simulink model "b6_formation"  (R2021b)
settings: Solver=FixedStepAuto  StartTime=0.0  StopTime=inf  FixedStep=sampleTime  RelTol=1e-3
PreLoadFcn:
  | % Simulation parameters
  | %load exampleMap
  | 
  | % Lidar parameters
  | sensorOffset = [0,0];
  | scanAngles = -pi/2:pi/6:pi/2;
  | maxRange = 0.3;
InitFcn:
  | sampleTime = 0.05;
  | nMedianSize=3;
  | % Robot parameters
  | wheelRadius = 0.0335;
  | robotRadius = 0.116/2;
  | 
  | %角速度坐标
  | ks=1;
  | 
  | % Lidar parameters
  | sensorOffset = [0,0];
  | scanAngles = -pi:pi/36:pi;
  | maxRange = 0.2;
  | 
  | %车初始位置
  | init_pose_1=[1  1.3  pi/2]';
  | init_pose_2=[0.85 1  pi/2]';
  | init_pose_3=[1.15 1  pi/2]';
  | init_pose_4=[0.7  0.7 pi/2]';
  | init_pose_5=[1  0.7 pi/2]';
  | init_pose_6=[1.3 0.7  pi/2]';
  | 
  | %pp算法性能参数
  | Vd_pp=0.2;
  | Wd_pp=pi;
  | dist_pp=0.2;
  | GoalRadius=0.1;
  | numSector=180;
  | rangeDis=[0.1,maxRange];
  | thresholds=[1/360 1/36];
  | safetyDis=0.2;
  | minimumTurningRadius=0.5*robotRadius;
  | recovery_w=0.05;
undefined symbols (not defined in the file): Angular, DiscIntNeverNeededParam, Linear, Pose, Twist
libraries: robotlib x42, dspstat3 x18, mobileRoboticsLib x7, robotmobilelib x6, robotalgslib x6
(part 1 of 5)
settings Model: Creator=FCS  LastModifiedBy=FCS

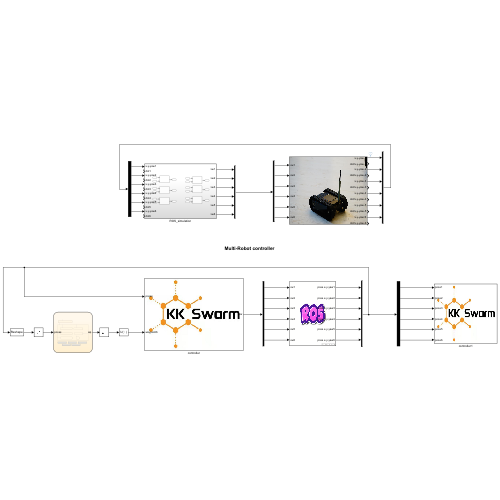
[thumbnail: Simulink's stored preview of the top-level diagram]
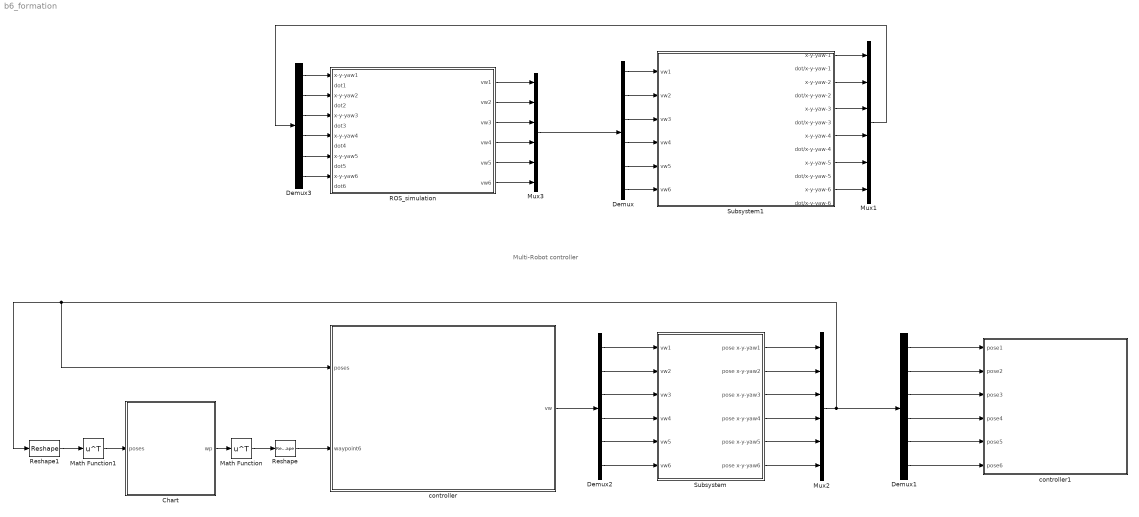
== system b6_formation ==
  note: Multi-Robot controller
  Chart : Stateflow chart  TreatAsAtomicUnit=on
  Demux{,1..3} (4 alike) : Demux  Outputs=6
  Math Function : Math  Operator=transpose  SaturateOnIntegerOverflow=on
  Math Function1 : Math  Operator=transpose  SaturateOnIntegerOverflow=on
  Mux1 : Mux  Inputs=6
  Mux2 : Mux  Inputs=6
  Mux3 : Mux  Inputs=6
  ROS_simulation : Subsystem
  Reshape : Reshape
  Reshape1 : Reshape  OutputDimensionality=Customize  OutputDimensions=[3,6]
  Subsystem : Subsystem
      mask Display: image('$imagefile'); % 使用工具条上的 "编辑图像" 进行更改。
  Subsystem1 : Subsystem
      mask Display: image('$imagefile'); % 使用工具条上的 "编辑图像" 进行更改。
  controller : Subsystem
      mask Display: image('$imagefile'); % 使用工具条上的 "编辑图像" 进行更改。
  controller1 : Subsystem
      mask Display: image('$imagefile'); % 使用工具条上的 "编辑图像" 进行更改。
  wires:
  Demux3/5 -> ROS_simulation/9(x-y-yaw5)
  Demux/3 -> Subsystem1/3(vw3)
  ROS_simulation/2(vw2) -> Mux3/2
  Demux3/1 -> ROS_simulation/1(x-y-yaw1)
  Subsystem1/9(x-y-yaw-5) -> Mux1/5
  Demux/2 -> Subsystem1/2(vw2)
  Demux/5 -> Subsystem1/5(vw5)
  Demux3/2 -> ROS_simulation/3(x-y-yaw2)
  Mux1/1 -> Demux3/1
  Subsystem1/1(x-y-yaw-1) -> Mux1/1
  ROS_simulation/5(vw5) -> Mux3/5
  Subsystem1/5(x-y-yaw-3) -> Mux1/3
  ROS_simulation/3(vw3) -> Mux3/3
  Subsystem1/7(x-y-yaw-4) -> Mux1/4
  Subsystem1/3(x-y-yaw-2) -> Mux1/2
  Demux3/4 -> ROS_simulation/7(x-y-yaw4)
  ROS_simulation/6(vw6) -> Mux3/6
  Demux/4 -> Subsystem1/4(vw4)
  ROS_simulation/4(vw4) -> Mux3/4
  Demux/1 -> Subsystem1/1(vw1)
  ROS_simulation/1(vw1) -> Mux3/1
  Subsystem1/11(x-y-yaw-6) -> Mux1/6
  Demux/6 -> Subsystem1/6(vw6)
  Mux3/1 -> Demux/1
  Demux3/3 -> ROS_simulation/5(x-y-yaw3)
  Demux3/6 -> ROS_simulation/11(x-y-yaw6)
  Subsystem/3(pose x-y-yaw3) -> Mux2/3
  Subsystem/6(pose x-y-yaw6) -> Mux2/6
  Subsystem/1(pose x-y-yaw1) -> Mux2/1
  Demux2/1 -> Subsystem/1(vw1)
  Demux2/2 -> Subsystem/2(vw2)
  Demux2/6 -> Subsystem/6(vw6)
  Demux2/4 -> Subsystem/4(vw4)
  Subsystem/4(pose x-y-yaw4) -> Mux2/4
  Demux2/3 -> Subsystem/3(vw3)
  Subsystem/2(pose x-y-yaw2) -> Mux2/2
  Subsystem/5(pose x-y-yaw5) -> Mux2/5
  Demux2/5 -> Subsystem/5(vw5)
  controller/1(vw) -> Demux2/1
  Chart/1(wp) -> Math Function/1
  Math Function/1 -> Reshape/1
  Reshape/1 -> controller/2(waypoint6)
  Reshape1/1 -> Math Function1/1
  Math Function1/1 -> Chart/1(poses)
  Mux2/1 -> Reshape1/1, controller/1(poses), Demux1/1
  Demux1/1 -> controller1/1(pose1)
  Demux1/2 -> controller1/2(pose2)
  Demux1/3 -> controller1/3(pose3)
  Demux1/4 -> controller1/4(pose4)
  Demux1/5 -> controller1/5(pose5)
  Demux1/6 -> controller1/6(pose6)

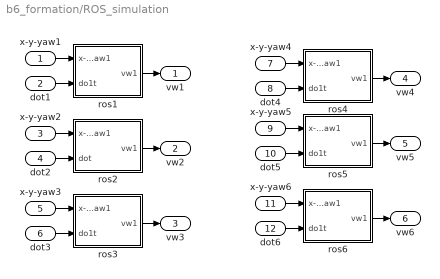
== system b6_formation/ROS_simulation ==
  x-y-yaw1 : Inport
  dot1 : Inport  Port=2
  x-y-yaw2 : Inport  Port=3
  dot2 : Inport  Port=4
  x-y-yaw3 : Inport  Port=5
  dot3 : Inport  Port=6
  x-y-yaw4 : Inport  Port=7
  dot4 : Inport  Port=8
  x-y-yaw5 : Inport  Port=9
  dot5 : Inport  Port=10
  x-y-yaw6 : Inport  Port=11
  dot6 : Inport  Port=12
  ros1 : Subsystem
  ros2 : Subsystem
  ros3 : Subsystem
  ros4 : Subsystem
  ros5 : Subsystem
  ros6 : Subsystem
  vw1 : Outport
  vw2 : Outport  Port=2
  vw3 : Outport  Port=3
  vw4 : Outport  Port=4
  vw5 : Outport  Port=5
  vw6 : Outport  Port=6
  wires:
  ros5/1(vw1) -> vw5/1
  ros2/1(vw1) -> vw2/1
  dot3/1 -> ros3/2(do1t)
  x-y-yaw5/1 -> ros5/1(x-y-yaw1)
  ros3/1(vw1) -> vw3/1
  dot2/1 -> ros2/2(dot)
  x-y-yaw2/1 -> ros2/1(x-y-yaw1)
  dot5/1 -> ros5/2(do1t)
  dot4/1 -> ros4/2(do1t)
  x-y-yaw4/1 -> ros4/1(x-y-yaw1)
  ros4/1(vw1) -> vw4/1
  x-y-yaw3/1 -> ros3/1(x-y-yaw1)
  dot6/1 -> ros6/2(do1t)
  x-y-yaw6/1 -> ros6/1(x-y-yaw1)
  dot1/1 -> ros1/2(do1t)
  ros6/1(vw1) -> vw6/1
  x-y-yaw1/1 -> ros1/1(x-y-yaw1)
  ros1/1(vw1) -> vw1/1

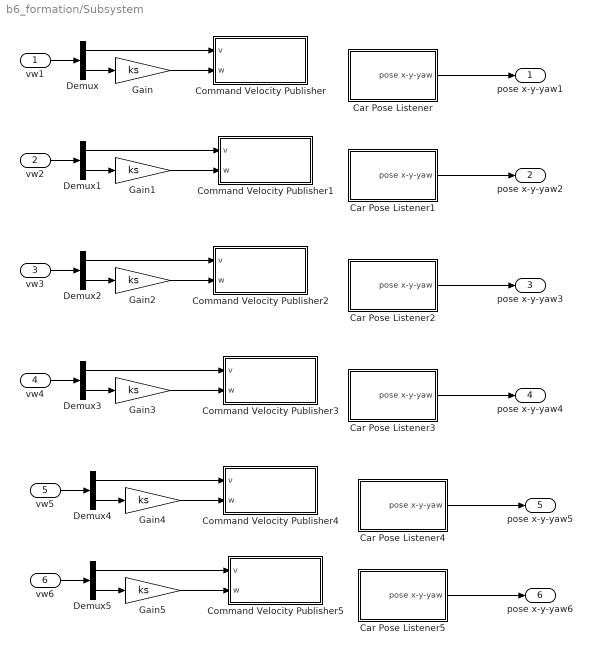
== system b6_formation/Subsystem ==
  vw1 : Inport
  vw2 : Inport  Port=2
  vw3 : Inport  Port=3
  vw4 : Inport  Port=4
  vw5 : Inport  Port=5
  vw6 : Inport  Port=6
  Car Pose Listener : Subsystem
  Car Pose Listener1 : Subsystem
  Car Pose Listener2 : Subsystem
  Car Pose Listener3 : Subsystem
  Car Pose Listener4 : Subsystem
  Car Pose Listener5 : Subsystem
  Command Velocity Publisher : Subsystem
  Command Velocity Publisher1 : Subsystem
  Command Velocity Publisher2 : Subsystem
  Command Velocity Publisher3 : Subsystem
  Command Velocity Publisher4 : Subsystem
  Command Velocity Publisher5 : Subsystem
  Demux{,1..5} (6 alike) : Demux  Outputs=2
  Gain{,1..5} (6 alike) : Gain  Gain=ks
  pose x-y-yaw1 : Outport
  pose x-y-yaw2 : Outport  Port=2
  pose x-y-yaw3 : Outport  Port=3
  pose x-y-yaw4 : Outport  Port=4
  pose x-y-yaw5 : Outport  Port=5
  pose x-y-yaw6 : Outport  Port=6
  wires:
  Gain/1 -> Command Velocity Publisher/2(w)
  Demux/2 -> Gain/1
  Car Pose Listener/1(pose x-y-yaw) -> pose x-y-yaw1/1
  Demux/1 -> Command Velocity Publisher/1(v)
  vw1/1 -> Demux/1
  Car Pose Listener1/1(pose x-y-yaw) -> pose x-y-yaw2/1
  Gain1/1 -> Command Velocity Publisher1/2(w)
  vw2/1 -> Demux1/1
  Demux1/2 -> Gain1/1
  Demux1/1 -> Command Velocity Publisher1/1(v)
  Car Pose Listener2/1(pose x-y-yaw) -> pose x-y-yaw3/1
  Gain2/1 -> Command Velocity Publisher2/2(w)
  vw3/1 -> Demux2/1
  Demux2/2 -> Gain2/1
  Demux2/1 -> Command Velocity Publisher2/1(v)
  Car Pose Listener3/1(pose x-y-yaw) -> pose x-y-yaw4/1
  Gain3/1 -> Command Velocity Publisher3/2(w)
  vw4/1 -> Demux3/1
  Demux3/2 -> Gain3/1
  Demux3/1 -> Command Velocity Publisher3/1(v)
  Car Pose Listener4/1(pose x-y-yaw) -> pose x-y-yaw5/1
  Gain4/1 -> Command Velocity Publisher4/2(w)
  vw5/1 -> Demux4/1
  Demux4/2 -> Gain4/1
  Car Pose Listener5/1(pose x-y-yaw) -> pose x-y-yaw6/1
  Gain5/1 -> Command Velocity Publisher5/2(w)
  vw6/1 -> Demux5/1
  Demux5/2 -> Gain5/1
  Demux5/1 -> Command Velocity Publisher5/1(v)
  Demux4/1 -> Command Velocity Publisher4/1(v)

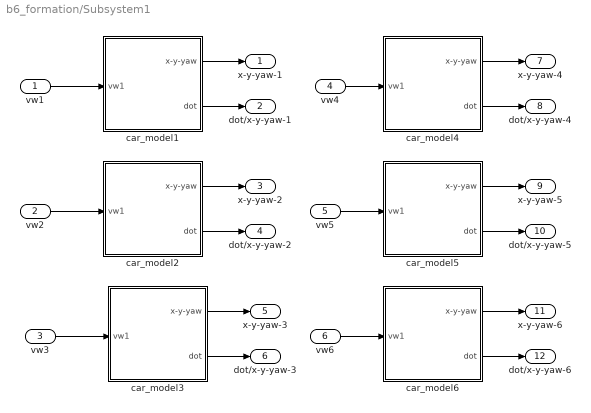
== system b6_formation/Subsystem1 ==
  vw1 : Inport
  vw2 : Inport  Port=2
  vw3 : Inport  Port=3
  vw4 : Inport  Port=4
  vw5 : Inport  Port=5
  vw6 : Inport  Port=6
  car_model1 : Subsystem
  car_model2 : Subsystem
  car_model3 : Subsystem
  car_model4 : Subsystem
  car_model5 : Subsystem
  car_model6 : Subsystem
  x-y-yaw-1 : Outport
  dot/x-y-yaw-1 : Outport  Port=2
  x-y-yaw-2 : Outport  Port=3
  dot/x-y-yaw-2 : Outport  Port=4
  x-y-yaw-3 : Outport  Port=5
  dot/x-y-yaw-3 : Outport  Port=6
  x-y-yaw-4 : Outport  Port=7
  dot/x-y-yaw-4 : Outport  Port=8
  x-y-yaw-5 : Outport  Port=9
  dot/x-y-yaw-5 : Outport  Port=10
  x-y-yaw-6 : Outport  Port=11
  dot/x-y-yaw-6 : Outport  Port=12
  wires:
  car_model1/1(x-y-yaw) -> x-y-yaw-1/1
  vw1/1 -> car_model1/1(vw1)
  car_model1/2(dot) -> dot/x-y-yaw-1/1
  car_model2/2(dot) -> dot/x-y-yaw-2/1
  vw2/1 -> car_model2/1(vw1)
  car_model2/1(x-y-yaw) -> x-y-yaw-2/1
  car_model3/1(x-y-yaw) -> x-y-yaw-3/1
  vw3/1 -> car_model3/1(vw1)
  car_model3/2(dot) -> dot/x-y-yaw-3/1
  car_model4/1(x-y-yaw) -> x-y-yaw-4/1
  vw4/1 -> car_model4/1(vw1)
  car_model4/2(dot) -> dot/x-y-yaw-4/1
  car_model5/1(x-y-yaw) -> x-y-yaw-5/1
  vw5/1 -> car_model5/1(vw1)
  car_model5/2(dot) -> dot/x-y-yaw-5/1
  car_model6/1(x-y-yaw) -> x-y-yaw-6/1
  vw6/1 -> car_model6/1(vw1)
  car_model6/2(dot) -> dot/x-y-yaw-6/1

== system b6_formation/controller ==
  poses : Inport
  waypoint6 : Inport  Port=2
  Car1 : Subsystem  mask{scanAngles=scanAngles, desired_v=Vd_pp, desired_w=Wd_pp, desired_lookahead=dist_pp, GoalRadius=GoalRadius, numSector=numSector, rangeDis=rangeDis, thresholds=thresholds, vehicleRadius=robotRadius, safetyDis=safetyDis, minimumTurningRadius=minimumTurningRadius, recovery_w=recovery_w}
      mask prompts: scanAngles "雷达扫描线角度"; desired_v "pp算法期望速度"; desired_w "pp算法期望角速度"; desired_lookahead "pp算法预瞄距离"; GoalRadius "到达目标的判定阈值"; numSector "直方图条柱数"; rangeDis "避障传感器距离范围"; thresholds "直方图障碍物占用空间阈值"; vehicleRadius "车辆半径"; safetyDis "车辆周边安全距离"; minimumTurningRadius "车辆的最少转弯半径"
  Car2 : Subsystem  mask{scanAngles=scanAngles, desired_v=Vd_pp, desired_w=Wd_pp, desired_lookahead=dist_pp, GoalRadius=GoalRadius, numSector=numSector, rangeDis=rangeDis, thresholds=thresholds, vehicleRadius=robotRadius, safetyDis=safetyDis, minimumTurningRadius=minimumTurningRadius, recovery_w=recovery_w}
      mask prompts: scanAngles "雷达扫描线角度"; desired_v "pp算法期望速度"; desired_w "pp算法期望角速度"; desired_lookahead "pp算法预瞄距离"; GoalRadius "到达目标的判定阈值"; numSector "直方图条柱数"; rangeDis "避障传感器距离范围"; thresholds "直方图障碍物占用空间阈值"; vehicleRadius "车辆半径"; safetyDis "车辆周边安全距离"; minimumTurningRadius "车辆的最少转弯半径"
  Car3 : Subsystem  mask{scanAngles=scanAngles, desired_v=Vd_pp, desired_w=Wd_pp, desired_lookahead=dist_pp, GoalRadius=GoalRadius, numSector=numSector, rangeDis=rangeDis, thresholds=thresholds, vehicleRadius=robotRadius, safetyDis=safetyDis, minimumTurningRadius=minimumTurningRadius, recovery_w=recovery_w}
      mask prompts: scanAngles "雷达扫描线角度"; desired_v "pp算法期望速度"; desired_w "pp算法期望角速度"; desired_lookahead "pp算法预瞄距离"; GoalRadius "到达目标的判定阈值"; numSector "直方图条柱数"; rangeDis "避障传感器距离范围"; thresholds "直方图障碍物占用空间阈值"; vehicleRadius "车辆半径"; safetyDis "车辆周边安全距离"; minimumTurningRadius "车辆的最少转弯半径"
  Car4 : Subsystem  mask{scanAngles=scanAngles, desired_v=Vd_pp, desired_w=Wd_pp, desired_lookahead=dist_pp, GoalRadius=GoalRadius, numSector=numSector, rangeDis=rangeDis, thresholds=thresholds, vehicleRadius=robotRadius, safetyDis=safetyDis, minimumTurningRadius=minimumTurningRadius, recovery_w=recovery_w}
      mask prompts: scanAngles "雷达扫描线角度"; desired_v "pp算法期望速度"; desired_w "pp算法期望角速度"; desired_lookahead "pp算法预瞄距离"; GoalRadius "到达目标的判定阈值"; numSector "直方图条柱数"; rangeDis "避障传感器距离范围"; thresholds "直方图障碍物占用空间阈值"; vehicleRadius "车辆半径"; safetyDis "车辆周边安全距离"; minimumTurningRadius "车辆的最少转弯半径"
  Car5 : Subsystem  mask{scanAngles=scanAngles, desired_v=Vd_pp, desired_w=Wd_pp, desired_lookahead=dist_pp, GoalRadius=GoalRadius, numSector=numSector, rangeDis=rangeDis, thresholds=thresholds, vehicleRadius=robotRadius, safetyDis=safetyDis, minimumTurningRadius=minimumTurningRadius, recovery_w=recovery_w}
      mask prompts: scanAngles "雷达扫描线角度"; desired_v "pp算法期望速度"; desired_w "pp算法期望角速度"; desired_lookahead "pp算法预瞄距离"; GoalRadius "到达目标的判定阈值"; numSector "直方图条柱数"; rangeDis "避障传感器距离范围"; thresholds "直方图障碍物占用空间阈值"; vehicleRadius "车辆半径"; safetyDis "车辆周边安全距离"; minimumTurningRadius "车辆的最少转弯半径"
  Car6 : Subsystem  mask{scanAngles=scanAngles, desired_v=Vd_pp, desired_w=Wd_pp, desired_lookahead=dist_pp, GoalRadius=GoalRadius, numSector=numSector, rangeDis=rangeDis, thresholds=thresholds, vehicleRadius=robotRadius, safetyDis=safetyDis, minimumTurningRadius=minimumTurningRadius, recovery_w=recovery_w}
      mask prompts: scanAngles "雷达扫描线角度"; desired_v "pp算法期望速度"; desired_w "pp算法期望角速度"; desired_lookahead "pp算法预瞄距离"; GoalRadius "到达目标的判定阈值"; numSector "直方图条柱数"; rangeDis "避障传感器距离范围"; thresholds "直方图障碍物占用空间阈值"; vehicleRadius "车辆半径"; safetyDis "车辆周边安全距离"; minimumTurningRadius "车辆的最少转弯半径"
  Demux : Demux  Outputs=6
  Demux1 : Demux  Outputs=6
  Mux : Mux  Inputs=6
  controller1 : Subsystem
      mask Display: image('$imagefile'); % 使用工具条上的 "编辑图像" 进行更改。
  vw : Outport
  wires:
  waypoint6/1 -> Demux1/1
  Mux/1 -> vw/1
  Car1/1(Out1) -> Mux/1
  poses/1 -> controller1/1(poses), Demux/1
  Car2/1(Out1) -> Mux/2
  Car6/1(Out1) -> Mux/6
  Car5/1(Out1) -> Mux/5
  Car4/1(Out1) -> Mux/4
  Car3/1(Out1) -> Mux/3
  Demux/1 -> Car1/2(Pose)
  Demux/2 -> Car2/2(Pose)
  Demux/3 -> Car3/2(Pose)
  Demux/4 -> Car4/2(Pose)
  Demux/5 -> Car5/2(Pose)
  Demux/6 -> Car6/2(Pose)
  Demux1/1 -> Car1/3(WayPoints)
  Demux1/2 -> Car2/3(WayPoints)
  Demux1/3 -> Car3/3(WayPoints)
  Demux1/4 -> Car4/3(WayPoints)
  Demux1/5 -> Car5/3(WayPoints)
  Demux1/6 -> Car6/3(WayPoints)
  controller1/1(Lidar1) -> Car1/1(Ranges)
  controller1/2(Lidar2) -> Car2/1(Ranges)
  controller1/3(Lidar3) -> Car3/1(Ranges)
  controller1/4(Lidar4) -> Car4/1(Ranges)
  controller1/5(Lidar5) -> Car5/1(Ranges)
  controller1/6(Lidar6) -> Car6/1(Ranges)

== system b6_formation/controller1 ==
  pose1 : Inport
  pose2 : Inport  Port=2
  pose3 : Inport  Port=3
  pose4 : Inport  Port=4
  pose5 : Inport  Port=5
  pose6 : Inport  Port=6
  Constant3 : Constant  Value="[0,0; 2,0;  2,2;  0,2]"
  Visualize Robot 1 : mobileRoboticsLib/Environments/Multi-Robot Visualizer  idx=1  radius=robotRadius  robotColor=[0 0 1]  showTraj=off  hasLidar=off  sensorOffset=sensorOffset  scanAngles=scanAngles  maxNumScans=0  hasObjDetector=off  objDetectorOffset=[0,0]  objDetectorAngle=0  objDetectorFOV=pi/2  objDetectorMaxRange=5  hasRobotDetector=off  robotDetectorOffset=[0,0]  robotDetectorAngle=0  robotDetectorFOV=pi/3  robotDetectorMaxRange=5  robotDetectorNumDetections=0
      settings: SourceProductName=Mobile Robotics Simulation Toolbox
  Visualize Robot 2 : mobileRoboticsLib/Environments/Multi-Robot Visualizer  idx=2  radius=robotRadius  robotColor=[0 1 0]  showTraj=on  hasLidar=off  sensorOffset=sensorOffset  scanAngles=scanAngles  maxNumScans=0  hasObjDetector=off  objDetectorOffset=[0,0]  objDetectorAngle=0  objDetectorFOV=pi/2  objDetectorMaxRange=5  hasRobotDetector=off  robotDetectorOffset=[0,0]  robotDetectorAngle=0  robotDetectorFOV=pi/3  robotDetectorMaxRange=5  robotDetectorNumDetections=0
      settings: SourceProductName=Mobile Robotics Simulation Toolbox
  Visualize Robot 3 : mobileRoboticsLib/Environments/Multi-Robot Visualizer  idx=3  radius=robotRadius  robotColor=[0 1 0]  showTraj=off  hasLidar=off  sensorOffset=sensorOffset  scanAngles=scanAngles  maxNumScans=0  hasObjDetector=off  objDetectorOffset=[0,0]  objDetectorAngle=0  objDetectorFOV=pi/2  objDetectorMaxRange=5  hasRobotDetector=off  robotDetectorOffset=[0,0]  robotDetectorAngle=0  robotDetectorFOV=pi/3  robotDetectorMaxRange=5  robotDetectorNumDetections=0
      settings: SourceProductName=Mobile Robotics Simulation Toolbox
  Visualize Robot 4 : mobileRoboticsLib/Environments/Multi-Robot Visualizer  idx=4  radius=robotRadius  robotColor=[1 0 0]  showTraj=on  hasLidar=off  sensorOffset=sensorOffset  scanAngles=scanAngles  maxNumScans=0  hasObjDetector=off  objDetectorOffset=[0,0]  objDetectorAngle=0  objDetectorFOV=pi/2  objDetectorMaxRange=5  hasRobotDetector=off  robotDetectorOffset=[0,0]  robotDetectorAngle=0  robotDetectorFOV=pi/3  robotDetectorMaxRange=5  robotDetectorNumDetections=0
      settings: SourceProductName=Mobile Robotics Simulation Toolbox
  Visualize Robot 5 : mobileRoboticsLib/Environments/Multi-Robot Visualizer  idx=5  radius=robotRadius  robotColor=[1 0 1]  showTraj=off  hasLidar=off  sensorOffset=sensorOffset  scanAngles=scanAngles  maxNumScans=0  hasObjDetector=off  objDetectorOffset=[0,0]  objDetectorAngle=0  objDetectorFOV=pi/2  objDetectorMaxRange=5  hasRobotDetector=off  robotDetectorOffset=[0,0]  robotDetectorAngle=0  robotDetectorFOV=pi/3  robotDetectorMaxRange=5  robotDetectorNumDetections=0
      settings: SourceProductName=Mobile Robotics Simulation Toolbox
  Visualize Robot 6 : mobileRoboticsLib/Environments/Multi-Robot Visualizer  idx=6  radius=robotRadius  robotColor=[1 0 0]  showTraj=off  hasLidar=off  sensorOffset=sensorOffset  scanAngles=scanAngles  maxNumScans=0  hasObjDetector=off  objDetectorOffset=[0,0]  objDetectorAngle=0  objDetectorFOV=pi/2  objDetectorMaxRange=5  hasRobotDetector=off  robotDetectorOffset=[0,0]  robotDetectorAngle=0  robotDetectorFOV=pi/3  robotDetectorMaxRange=5  robotDetectorNumDetections=0
      settings: SourceProductName=Mobile Robotics Simulation Toolbox
  World1 : mobileRoboticsLib/Environments/Multi-Robot Environment  numRobots=6  showWaypoints=on  showObjects=off  objectColors=[1 0 0;0 1 0;0 0 1]  objectMarkers='s'  showRobotIds=on  plotSensorLines=on
      settings: SourceProductName=Mobile Robotics Simulation Toolbox
  wires:
  pose2/1 -> Visualize Robot 2/1
  pose6/1 -> Visualize Robot 6/1
  pose1/1 -> Visualize Robot 1/1
  pose4/1 -> Visualize Robot 4/1
  pose5/1 -> Visualize Robot 5/1
  pose3/1 -> Visualize Robot 3/1
  Constant3/1 -> World1/1

== system b6_formation/ROS_simulation/ros1 ==
  x-y-yaw1 : Inport
  do1t : Inport  Port=2
  " [x y theta]" : Demux  Outputs=3
  " [x y theta]1" : Demux  Outputs=3
  Blank Message : robotlib/Blank Message  messageClass=Message  entityType=nav_msgs/Odometry  messageType=nav_msgs/Odometry  SampleTime=inf  legacyBusStruct=off
  Bus Assignment1 : BusAssignment  DialogController=Simulink.DDGSource_BusAssignment  AssignedSignals=Pose.Pose.Position.X,Pose.Pose.Position.Y,Pose.Pose.Orientation.Z,Pose.Pose.Orientation.W,Twist.Twist.Linear.X,Twist.Twist.Linear.Y,Twist.Twist.Angular.Z
  MATLAB Function : MATLAB Function  TreatAsAtomicUnit=on
  MATLAB Function3 : MATLAB Function  TreatAsAtomicUnit=on
  Mux6 : Mux  Inputs=2
  Publish2 : robotlib/Publish  topicSource=Specify your own  topic=/robot_1/pose  messageType=nav_msgs/Odometry  legacyBusStruct=off  messageQueueLength=105
  Subscribe1 : robotlib/Subscribe  topicSource=Specify your own  topic=/robot_1/cmd_vel  messageType=geometry_msgs/Twist  SampleTime=-1  legacyBusStruct=off  messageQueueLength=51
  Terminator : Terminator
  Terminator1 : Terminator
  Zero-Order Hold : ZeroOrderHold  SampleTime=0.1
  Zero-Order Hold1 : ZeroOrderHold  SampleTime=0.1
  vw1 : Outport
  wires:
  " [x y theta]"/1 -> Bus Assignment1/2
  Blank Message/1 -> Bus Assignment1/1
  x-y-yaw1/1 -> Zero-Order Hold/1
  " [x y theta]"/2 -> Bus Assignment1/3
  " [x y theta]1"/2 -> Bus Assignment1/7
  " [x y theta]"/3 -> MATLAB Function/1(yaw)
  " [x y theta]1"/3 -> Bus Assignment1/8
  MATLAB Function/4(w) -> Bus Assignment1/5
  MATLAB Function/3(z) -> Bus Assignment1/4
  " [x y theta]1"/1 -> Bus Assignment1/6
  Bus Assignment1/1 -> Publish2/1
  do1t/1 -> Zero-Order Hold1/1
  MATLAB Function/1(x) -> Terminator/1
  MATLAB Function/2(y) -> Terminator1/1
  Zero-Order Hold/1 -> " [x y theta]"/1
  Zero-Order Hold1/1 -> " [x y theta]1"/1
  Mux6/1 -> vw1/1
  MATLAB Function3/2(wref) -> Mux6/2
  MATLAB Function3/1(vref) -> Mux6/1
  Subscribe1/1 -> MATLAB Function3/1(IsNew)
  Subscribe1/2 -> MATLAB Function3/2(cmdMsg)

== system b6_formation/ROS_simulation/ros2 ==
  x-y-yaw1 : Inport
  dot : Inport  Port=2
  " [x y theta]" : Demux  Outputs=3
  " [x y theta]1" : Demux  Outputs=3
  Blank Message : robotlib/Blank Message  messageClass=Message  entityType=nav_msgs/Odometry  messageType=nav_msgs/Odometry  SampleTime=inf  legacyBusStruct=off
  Bus Assignment1 : BusAssignment  DialogController=Simulink.DDGSource_BusAssignment  AssignedSignals=Pose.Pose.Position.X,Pose.Pose.Position.Y,Pose.Pose.Orientation.Z,Pose.Pose.Orientation.W,Twist.Twist.Linear.X,Twist.Twist.Linear.Y,Twist.Twist.Angular.Z
  MATLAB Function : MATLAB Function  TreatAsAtomicUnit=on
  MATLAB Function3 : MATLAB Function  TreatAsAtomicUnit=on
  Mux6 : Mux  Inputs=2
  Publish2 : robotlib/Publish  topicSource=Specify your own  topic=/robot_2/pose  messageType=nav_msgs/Odometry  legacyBusStruct=off  messageQueueLength=105
  Subscribe1 : robotlib/Subscribe  topicSource=Specify your own  topic=/robot_2/cmd_vel  messageType=geometry_msgs/Twist  SampleTime=-1  legacyBusStruct=off  messageQueueLength=51
  Terminator : Terminator
  Terminator1 : Terminator
  Zero-Order Hold : ZeroOrderHold  SampleTime=0.1
  Zero-Order Hold1 : ZeroOrderHold  SampleTime=0.1
  vw1 : Outport
  wires:
  " [x y theta]"/1 -> Bus Assignment1/2
  Blank Message/1 -> Bus Assignment1/1
  x-y-yaw1/1 -> Zero-Order Hold/1
  " [x y theta]"/2 -> Bus Assignment1/3
  " [x y theta]1"/2 -> Bus Assignment1/7
  " [x y theta]"/3 -> MATLAB Function/1(yaw)
  " [x y theta]1"/3 -> Bus Assignment1/8
  MATLAB Function/4(w) -> Bus Assignment1/5
  MATLAB Function/3(z) -> Bus Assignment1/4
  " [x y theta]1"/1 -> Bus Assignment1/6
  Bus Assignment1/1 -> Publish2/1
  dot/1 -> Zero-Order Hold1/1
  MATLAB Function/1(x) -> Terminator/1
  MATLAB Function/2(y) -> Terminator1/1
  Zero-Order Hold/1 -> " [x y theta]"/1
  Zero-Order Hold1/1 -> " [x y theta]1"/1
  MATLAB Function3/1(vref) -> Mux6/1
  MATLAB Function3/2(wref) -> Mux6/2
  Subscribe1/1 -> MATLAB Function3/1(IsNew)
  Subscribe1/2 -> MATLAB Function3/2(cmdMsg)
  Mux6/1 -> vw1/1

== system b6_formation/ROS_simulation/ros3 ==
  x-y-yaw1 : Inport
  do1t : Inport  Port=2
  " [x y theta]" : Demux  Outputs=3
  " [x y theta]1" : Demux  Outputs=3
  Blank Message : robotlib/Blank Message  messageClass=Message  entityType=nav_msgs/Odometry  messageType=nav_msgs/Odometry  SampleTime=inf  legacyBusStruct=off
  Bus Assignment1 : BusAssignment  DialogController=Simulink.DDGSource_BusAssignment  AssignedSignals=Pose.Pose.Position.X,Pose.Pose.Position.Y,Pose.Pose.Orientation.Z,Pose.Pose.Orientation.W,Twist.Twist.Linear.X,Twist.Twist.Linear.Y,Twist.Twist.Angular.Z
  MATLAB Function : MATLAB Function  TreatAsAtomicUnit=on
  MATLAB Function3 : MATLAB Function  TreatAsAtomicUnit=on
  Mux6 : Mux  Inputs=2
  Publish2 : robotlib/Publish  topicSource=Specify your own  topic=/robot_3/pose  messageType=nav_msgs/Odometry  legacyBusStruct=off  messageQueueLength=105
  Subscribe1 : robotlib/Subscribe  topicSource=Specify your own  topic=/robot_3/cmd_vel  messageType=geometry_msgs/Twist  SampleTime=-1  legacyBusStruct=off  messageQueueLength=51
  Terminator : Terminator
  Terminator1 : Terminator
  Zero-Order Hold : ZeroOrderHold  SampleTime=0.1
  Zero-Order Hold1 : ZeroOrderHold  SampleTime=0.1
  vw1 : Outport
  wires:
  " [x y theta]"/1 -> Bus Assignment1/2
  Blank Message/1 -> Bus Assignment1/1
  x-y-yaw1/1 -> Zero-Order Hold/1
  " [x y theta]"/2 -> Bus Assignment1/3
  " [x y theta]1"/2 -> Bus Assignment1/7
  " [x y theta]"/3 -> MATLAB Function/1(yaw)
  " [x y theta]1"/3 -> Bus Assignment1/8
  MATLAB Function/4(w) -> Bus Assignment1/5
  MATLAB Function/3(z) -> Bus Assignment1/4
  " [x y theta]1"/1 -> Bus Assignment1/6
  Bus Assignment1/1 -> Publish2/1
  do1t/1 -> Zero-Order Hold1/1
  MATLAB Function/1(x) -> Terminator/1
  MATLAB Function/2(y) -> Terminator1/1
  Zero-Order Hold/1 -> " [x y theta]"/1
  Zero-Order Hold1/1 -> " [x y theta]1"/1
  MATLAB Function3/1(vref) -> Mux6/1
  MATLAB Function3/2(wref) -> Mux6/2
  Subscribe1/1 -> MATLAB Function3/1(IsNew)
  Subscribe1/2 -> MATLAB Function3/2(cmdMsg)
  Mux6/1 -> vw1/1

== system b6_formation/ROS_simulation/ros4 ==
  x-y-yaw1 : Inport
  do1t : Inport  Port=2
  " [x y theta]" : Demux  Outputs=3
  " [x y theta]1" : Demux  Outputs=3
  Blank Message : robotlib/Blank Message  messageClass=Message  entityType=nav_msgs/Odometry  messageType=nav_msgs/Odometry  SampleTime=inf  legacyBusStruct=off
  Bus Assignment1 : BusAssignment  DialogController=Simulink.DDGSource_BusAssignment  AssignedSignals=Pose.Pose.Position.X,Pose.Pose.Position.Y,Pose.Pose.Orientation.Z,Pose.Pose.Orientation.W,Twist.Twist.Linear.X,Twist.Twist.Linear.Y,Twist.Twist.Angular.Z
  MATLAB Function : MATLAB Function  TreatAsAtomicUnit=on
  MATLAB Function3 : MATLAB Function  TreatAsAtomicUnit=on
  Mux6 : Mux  Inputs=2
  Publish2 : robotlib/Publish  topicSource=Specify your own  topic=/robot_4/pose  messageType=nav_msgs/Odometry  legacyBusStruct=off  messageQueueLength=105
  Subscribe1 : robotlib/Subscribe  topicSource=Specify your own  topic=/robot_4/cmd_vel  messageType=geometry_msgs/Twist  SampleTime=-1  legacyBusStruct=off  messageQueueLength=51
  Terminator : Terminator
  Terminator1 : Terminator
  Zero-Order Hold : ZeroOrderHold  SampleTime=0.1
  Zero-Order Hold1 : ZeroOrderHold  SampleTime=0.1
  vw1 : Outport
  wires:
  " [x y theta]"/1 -> Bus Assignment1/2
  Blank Message/1 -> Bus Assignment1/1
  x-y-yaw1/1 -> Zero-Order Hold/1
  " [x y theta]"/2 -> Bus Assignment1/3
  " [x y theta]1"/2 -> Bus Assignment1/7
  " [x y theta]"/3 -> MATLAB Function/1(yaw)
  " [x y theta]1"/3 -> Bus Assignment1/8
  MATLAB Function/4(w) -> Bus Assignment1/5
  MATLAB Function/3(z) -> Bus Assignment1/4
  " [x y theta]1"/1 -> Bus Assignment1/6
  Bus Assignment1/1 -> Publish2/1
  do1t/1 -> Zero-Order Hold1/1
  MATLAB Function/1(x) -> Terminator/1
  MATLAB Function/2(y) -> Terminator1/1
  Zero-Order Hold/1 -> " [x y theta]"/1
  Zero-Order Hold1/1 -> " [x y theta]1"/1
  MATLAB Function3/1(vref) -> Mux6/1
  MATLAB Function3/2(wref) -> Mux6/2
  Subscribe1/1 -> MATLAB Function3/1(IsNew)
  Subscribe1/2 -> MATLAB Function3/2(cmdMsg)
  Mux6/1 -> vw1/1

== system b6_formation/ROS_simulation/ros5 ==
  x-y-yaw1 : Inport
  do1t : Inport  Port=2
  " [x y theta]" : Demux  Outputs=3
  " [x y theta]1" : Demux  Outputs=3
  Blank Message : robotlib/Blank Message  messageClass=Message  entityType=nav_msgs/Odometry  messageType=nav_msgs/Odometry  SampleTime=inf  legacyBusStruct=off
  Bus Assignment1 : BusAssignment  DialogController=Simulink.DDGSource_BusAssignment  AssignedSignals=Pose.Pose.Position.X,Pose.Pose.Position.Y,Pose.Pose.Orientation.Z,Pose.Pose.Orientation.W,Twist.Twist.Linear.X,Twist.Twist.Linear.Y,Twist.Twist.Angular.Z
  MATLAB Function : MATLAB Function  TreatAsAtomicUnit=on
  MATLAB Function3 : MATLAB Function  TreatAsAtomicUnit=on
  Mux6 : Mux  Inputs=2
  Publish2 : robotlib/Publish  topicSource=Specify your own  topic=/robot_5/pose  messageType=nav_msgs/Odometry  legacyBusStruct=off  messageQueueLength=105
  Subscribe1 : robotlib/Subscribe  topicSource=Specify your own  topic=/robot_5/cmd_vel  messageType=geometry_msgs/Twist  SampleTime=-1  legacyBusStruct=off  messageQueueLength=51
  Terminator : Terminator
  Terminator1 : Terminator
  Zero-Order Hold : ZeroOrderHold  SampleTime=0.1
  Zero-Order Hold1 : ZeroOrderHold  SampleTime=0.1
  vw1 : Outport
  wires:
  " [x y theta]"/1 -> Bus Assignment1/2
  Blank Message/1 -> Bus Assignment1/1
  x-y-yaw1/1 -> Zero-Order Hold/1
  " [x y theta]"/2 -> Bus Assignment1/3
  " [x y theta]1"/2 -> Bus Assignment1/7
  " [x y theta]"/3 -> MATLAB Function/1(yaw)
  " [x y theta]1"/3 -> Bus Assignment1/8
  MATLAB Function/4(w) -> Bus Assignment1/5
  MATLAB Function/3(z) -> Bus Assignment1/4
  " [x y theta]1"/1 -> Bus Assignment1/6
  Bus Assignment1/1 -> Publish2/1
  do1t/1 -> Zero-Order Hold1/1
  MATLAB Function/1(x) -> Terminator/1
  MATLAB Function/2(y) -> Terminator1/1
  Zero-Order Hold/1 -> " [x y theta]"/1
  Zero-Order Hold1/1 -> " [x y theta]1"/1
  MATLAB Function3/1(vref) -> Mux6/1
  MATLAB Function3/2(wref) -> Mux6/2
  Subscribe1/1 -> MATLAB Function3/1(IsNew)
  Subscribe1/2 -> MATLAB Function3/2(cmdMsg)
  Mux6/1 -> vw1/1

== system b6_formation/ROS_simulation/ros6 ==
  x-y-yaw1 : Inport
  do1t : Inport  Port=2
  " [x y theta]" : Demux  Outputs=3
  " [x y theta]1" : Demux  Outputs=3
  Blank Message : robotlib/Blank Message  messageClass=Message  entityType=nav_msgs/Odometry  messageType=nav_msgs/Odometry  SampleTime=inf  legacyBusStruct=off
  Bus Assignment1 : BusAssignment  DialogController=Simulink.DDGSource_BusAssignment  AssignedSignals=Pose.Pose.Position.X,Pose.Pose.Position.Y,Pose.Pose.Orientation.Z,Pose.Pose.Orientation.W,Twist.Twist.Linear.X,Twist.Twist.Linear.Y,Twist.Twist.Angular.Z
  MATLAB Function : MATLAB Function  TreatAsAtomicUnit=on
  MATLAB Function3 : MATLAB Function  TreatAsAtomicUnit=on
  Mux6 : Mux  Inputs=2
  Publish2 : robotlib/Publish  topicSource=Specify your own  topic=/robot_6/pose  messageType=nav_msgs/Odometry  legacyBusStruct=off  messageQueueLength=105
  Subscribe1 : robotlib/Subscribe  topicSource=Specify your own  topic=/robot_6/cmd_vel  messageType=geometry_msgs/Twist  SampleTime=-1  legacyBusStruct=off  messageQueueLength=51
  Terminator : Terminator
  Terminator1 : Terminator
  Zero-Order Hold : ZeroOrderHold  SampleTime=0.1
  Zero-Order Hold1 : ZeroOrderHold  SampleTime=0.1
  vw1 : Outport
  wires:
  " [x y theta]"/1 -> Bus Assignment1/2
  Blank Message/1 -> Bus Assignment1/1
  x-y-yaw1/1 -> Zero-Order Hold/1
  " [x y theta]"/2 -> Bus Assignment1/3
  " [x y theta]1"/2 -> Bus Assignment1/7
  " [x y theta]"/3 -> MATLAB Function/1(yaw)
  " [x y theta]1"/3 -> Bus Assignment1/8
  MATLAB Function/4(w) -> Bus Assignment1/5
  MATLAB Function/3(z) -> Bus Assignment1/4
  " [x y theta]1"/1 -> Bus Assignment1/6
  Bus Assignment1/1 -> Publish2/1
  do1t/1 -> Zero-Order Hold1/1
  MATLAB Function/1(x) -> Terminator/1
  MATLAB Function/2(y) -> Terminator1/1
  MATLAB Function3/1(vref) -> Mux6/1
  MATLAB Function3/2(wref) -> Mux6/2
  Subscribe1/1 -> MATLAB Function3/1(IsNew)
  Subscribe1/2 -> MATLAB Function3/2(cmdMsg)
  Mux6/1 -> vw1/1
  Zero-Order Hold/1 -> " [x y theta]"/1
  Zero-Order Hold1/1 -> " [x y theta]1"/1

== system b6_formation/Subsystem/Car Pose Listener ==
  Subscribe : robotlib/Subscribe  topicSource=Specify your own  topic=/robot_1/pose  messageType=nav_msgs/Odometry  SampleTime=-1  legacyBusStruct=off  messageQueueLength=51
  Subscribe1 : robotlib/Subscribe  topicSource=Specify your own  topic=/robot_1/odometry  messageType=geometry_msgs/Twist  SampleTime=-1  legacyBusStruct=off  messageQueueLength=51
  Subsystem : Subsystem
  pose x-y-yaw : Outport
  wires:
  Subscribe/1 -> Subsystem/1(poseNew)  "IsNew"
  Subscribe/2 -> Subsystem/2(poseMsg)
  Subscribe1/1 -> Subsystem/3(VW_New)  "IsNew"
  Subscribe1/2 -> Subsystem/4(VW_Msg)
  Subsystem/1(pose) -> pose x-y-yaw/1

== system b6_formation/Subsystem/Car Pose Listener1 ==
  Subscribe : robotlib/Subscribe  topicSource=Specify your own  topic=/robot_2/pose  messageType=nav_msgs/Odometry  SampleTime=-1  legacyBusStruct=off  messageQueueLength=51
  Subscribe1 : robotlib/Subscribe  topicSource=Specify your own  topic=/robot_2/odometry  messageType=geometry_msgs/Twist  SampleTime=-1  legacyBusStruct=off  messageQueueLength=51
  Subsystem : Subsystem
  pose x-y-yaw : Outport
  wires:
  Subscribe/1 -> Subsystem/1(poseNew)  "IsNew"
  Subscribe/2 -> Subsystem/2(poseMsg)
  Subscribe1/2 -> Subsystem/4(VW_Msg)
  Subscribe1/1 -> Subsystem/3(VW_New)  "IsNew"
  Subsystem/1(pose) -> pose x-y-yaw/1

== system b6_formation/Subsystem/Car Pose Listener2 ==
  Subscribe : robotlib/Subscribe  topicSource=Specify your own  topic=/robot_3/pose  messageType=nav_msgs/Odometry  SampleTime=-1  legacyBusStruct=off  messageQueueLength=51
  Subscribe1 : robotlib/Subscribe  topicSource=Specify your own  topic=/robot_3/odometry  messageType=geometry_msgs/Twist  SampleTime=-1  legacyBusStruct=off  messageQueueLength=51
  Subsystem : Subsystem
  pose x-y-yaw : Outport
  wires:
  Subscribe/1 -> Subsystem/1(poseNew)  "IsNew"
  Subscribe/2 -> Subsystem/2(poseMsg)
  Subscribe1/1 -> Subsystem/3(VW_New)  "IsNew"
  Subscribe1/2 -> Subsystem/4(VW_Msg)
  Subsystem/1(pose) -> pose x-y-yaw/1

== system b6_formation/Subsystem/Car Pose Listener3 ==
  Subscribe : robotlib/Subscribe  topicSource=Specify your own  topic=/robot_4/pose  messageType=nav_msgs/Odometry  SampleTime=-1  legacyBusStruct=off  messageQueueLength=51
  Subscribe1 : robotlib/Subscribe  topicSource=Specify your own  topic=/robot_4/odometry  messageType=geometry_msgs/Twist  SampleTime=-1  legacyBusStruct=off  messageQueueLength=51
  Subsystem : Subsystem
  pose x-y-yaw : Outport
  wires:
  Subscribe/1 -> Subsystem/1(poseNew)  "IsNew"
  Subscribe/2 -> Subsystem/2(poseMsg)
  Subscribe1/1 -> Subsystem/3(VW_New)  "IsNew"
  Subscribe1/2 -> Subsystem/4(VW_Msg)
  Subsystem/1(pose) -> pose x-y-yaw/1

== system b6_formation/Subsystem/Car Pose Listener4 ==
  Subscribe : robotlib/Subscribe  topicSource=Specify your own  topic=/robot_5/pose  messageType=nav_msgs/Odometry  SampleTime=-1  legacyBusStruct=off  messageQueueLength=51
  Subscribe1 : robotlib/Subscribe  topicSource=Specify your own  topic=/robot_5/odometry  messageType=geometry_msgs/Twist  SampleTime=-1  legacyBusStruct=off  messageQueueLength=51
  Subsystem : Subsystem
  pose x-y-yaw : Outport
  wires:
  Subscribe/1 -> Subsystem/1(poseNew)  "IsNew"
  Subscribe/2 -> Subsystem/2(poseMsg)
  Subscribe1/1 -> Subsystem/3(VW_New)  "IsNew"
  Subscribe1/2 -> Subsystem/4(VW_Msg)
  Subsystem/1(pose) -> pose x-y-yaw/1

== system b6_formation/Subsystem/Car Pose Listener5 ==
  Subscribe : robotlib/Subscribe  topicSource=Specify your own  topic=/robot_6/pose  messageType=nav_msgs/Odometry  SampleTime=-1  legacyBusStruct=off  messageQueueLength=51
  Subscribe1 : robotlib/Subscribe  topicSource=Specify your own  topic=/robot_6/odometry  messageType=geometry_msgs/Twist  SampleTime=-1  legacyBusStruct=off  messageQueueLength=51
  Subsystem : Subsystem
  pose x-y-yaw : Outport
  wires:
  Subscribe/1 -> Subsystem/1(poseNew)  "IsNew"
  Subscribe/2 -> Subsystem/2(poseMsg)
  Subscribe1/1 -> Subsystem/3(VW_New)  "IsNew"
  Subscribe1/2 -> Subsystem/4(VW_Msg)
  Subsystem/1(pose) -> pose x-y-yaw/1

== system b6_formation/Subsystem/Command Velocity Publisher ==
  v : Inport
  w : Inport  Port=2
  Blank Message : robotlib/Blank Message  messageClass=Message  entityType=geometry_msgs/Twist  messageType=geometry_msgs/Twist  SampleTime=inf  legacyBusStruct=off
  Bus Assignment1 : BusAssignment  DialogController=Simulink.DDGSource_BusAssignment  AssignedSignals=Linear.X,Angular.Z
  Publish2 : robotlib/Publish  topicSource=Specify your own  topic=/robot_1/cmd_vel  messageType=geometry_msgs/Twist  legacyBusStruct=off  messageQueueLength=105
  wires:
  Bus Assignment1/1 -> Publish2/1
  Blank Message/1 -> Bus Assignment1/1
  v/1 -> Bus Assignment1/2
  w/1 -> Bus Assignment1/3

== system b6_formation/Subsystem/Command Velocity Publisher1 ==
  v : Inport
  w : Inport  Port=2
  Blank Message : robotlib/Blank Message  messageClass=Message  entityType=geometry_msgs/Twist  messageType=geometry_msgs/Twist  SampleTime=inf  legacyBusStruct=off
  Bus Assignment1 : BusAssignment  DialogController=Simulink.DDGSource_BusAssignment  AssignedSignals=Linear.X,Angular.Z
  Publish2 : robotlib/Publish  topicSource=Specify your own  topic=/robot_2/cmd_vel  messageType=geometry_msgs/Twist  legacyBusStruct=off  messageQueueLength=105
  wires:
  Bus Assignment1/1 -> Publish2/1
  Blank Message/1 -> Bus Assignment1/1
  v/1 -> Bus Assignment1/2
  w/1 -> Bus Assignment1/3

== system b6_formation/Subsystem/Command Velocity Publisher2 ==
  v : Inport
  w : Inport  Port=2
  Blank Message : robotlib/Blank Message  messageClass=Message  entityType=geometry_msgs/Twist  messageType=geometry_msgs/Twist  SampleTime=inf  legacyBusStruct=off
  Bus Assignment1 : BusAssignment  DialogController=Simulink.DDGSource_BusAssignment  AssignedSignals=Linear.X,Angular.Z
  Publish2 : robotlib/Publish  topicSource=Specify your own  topic=/robot_3/cmd_vel  messageType=geometry_msgs/Twist  legacyBusStruct=off  messageQueueLength=105
  wires:
  Bus Assignment1/1 -> Publish2/1
  Blank Message/1 -> Bus Assignment1/1
  v/1 -> Bus Assignment1/2
  w/1 -> Bus Assignment1/3

== system b6_formation/Subsystem/Command Velocity Publisher3 ==
  v : Inport
  w : Inport  Port=2
  Blank Message : robotlib/Blank Message  messageClass=Message  entityType=geometry_msgs/Twist  messageType=geometry_msgs/Twist  SampleTime=inf  legacyBusStruct=off
  Bus Assignment1 : BusAssignment  DialogController=Simulink.DDGSource_BusAssignment  AssignedSignals=Linear.X,Angular.Z
  Publish2 : robotlib/Publish  topicSource=Specify your own  topic=/robot_4/cmd_vel  messageType=geometry_msgs/Twist  legacyBusStruct=off  messageQueueLength=105
  wires:
  Bus Assignment1/1 -> Publish2/1
  Blank Message/1 -> Bus Assignment1/1
  v/1 -> Bus Assignment1/2
  w/1 -> Bus Assignment1/3

== system b6_formation/Subsystem/Command Velocity Publisher4 ==
  v : Inport
  w : Inport  Port=2
  Blank Message : robotlib/Blank Message  messageClass=Message  entityType=geometry_msgs/Twist  messageType=geometry_msgs/Twist  SampleTime=inf  legacyBusStruct=off
  Bus Assignment1 : BusAssignment  DialogController=Simulink.DDGSource_BusAssignment  AssignedSignals=Linear.X,Angular.Z
  Publish2 : robotlib/Publish  topicSource=Specify your own  topic=/robot_5/cmd_vel  messageType=geometry_msgs/Twist  legacyBusStruct=off  messageQueueLength=105
  wires:
  Bus Assignment1/1 -> Publish2/1
  Blank Message/1 -> Bus Assignment1/1
  v/1 -> Bus Assignment1/2
  w/1 -> Bus Assignment1/3

== system b6_formation/Subsystem/Command Velocity Publisher5 ==
  v : Inport
  w : Inport  Port=2
  Blank Message : robotlib/Blank Message  messageClass=Message  entityType=geometry_msgs/Twist  messageType=geometry_msgs/Twist  SampleTime=inf  legacyBusStruct=off
  Bus Assignment1 : BusAssignment  DialogController=Simulink.DDGSource_BusAssignment  AssignedSignals=Linear.X,Angular.Z
  Publish2 : robotlib/Publish  topicSource=Specify your own  topic=/robot_6/cmd_vel  messageType=geometry_msgs/Twist  legacyBusStruct=off  messageQueueLength=105
  wires:
  Bus Assignment1/1 -> Publish2/1
  Blank Message/1 -> Bus Assignment1/1
  v/1 -> Bus Assignment1/2
  w/1 -> Bus Assignment1/3

== system b6_formation/Subsystem1/car_model1 ==
  note: tr=0.6
      | 4T=0.6
      | 一阶系统的动态性能指标为：td=0.69T，tr=2.20T，ts=3T
  vw1 : Inport
  Demux : Demux  Outputs=2
  Differential Drive Kinematic Model1 : robotmobilelib/Differential Drive Kinematic Model  VehicleInputs=Vehicle Speed & Heading Angular Velocity  WheelRadius=wheelRadius  WheelSpeedRange=[-inf inf]  TrackWidth=robotRadius  InitialState=init_pose_1  SimulateUsing=Interpreted execution
      settings: SourceProductBaseCode=RO
  Simulink顺时针为正 小车逆时针为正 : Gain  Gain=ks
  Transfer Fcn : TransferFcn  Denominator=[0.15 1]
  Transfer Fcn1 : TransferFcn  Denominator=[0.16 1]
  x-y-yaw : Outport
  dot : Outport  Port=2
  wires:
  Simulink顺时针为正 小车逆时针为正/1 -> Transfer Fcn1/1
  Transfer Fcn/1 -> Differential Drive Kinematic Model1/1
  Demux/1 -> Transfer Fcn/1
  Transfer Fcn1/1 -> Differential Drive Kinematic Model1/2
  Demux/2 -> Simulink顺时针为正 小车逆时针为正/1
  vw1/1 -> Demux/1
  Differential Drive Kinematic Model1/1 -> x-y-yaw/1
  Differential Drive Kinematic Model1/2 -> dot/1

== system b6_formation/Subsystem1/car_model2 ==
  note: tr=0.6
      | 4T=0.6
      | 一阶系统的动态性能指标为：td=0.69T，tr=2.20T，ts=3T
  vw1 : Inport
  Demux : Demux  Outputs=2
  Differential Drive Kinematic Model1 : robotmobilelib/Differential Drive Kinematic Model  VehicleInputs=Vehicle Speed & Heading Angular Velocity  WheelRadius=wheelRadius  WheelSpeedRange=[-inf inf]  TrackWidth=robotRadius  InitialState=init_pose_2  SimulateUsing=Interpreted execution
      settings: SourceProductBaseCode=RO
  Simulink顺时针为正 小车逆时针为正 : Gain  Gain=ks
  Transfer Fcn : TransferFcn  Denominator=[0.15 1]
  Transfer Fcn1 : TransferFcn  Denominator=[0.16 1]
  x-y-yaw : Outport
  dot : Outport  Port=2
  wires:
  Simulink顺时针为正 小车逆时针为正/1 -> Transfer Fcn1/1
  Transfer Fcn/1 -> Differential Drive Kinematic Model1/1
  Demux/1 -> Transfer Fcn/1
  Transfer Fcn1/1 -> Differential Drive Kinematic Model1/2
  Demux/2 -> Simulink顺时针为正 小车逆时针为正/1
  vw1/1 -> Demux/1
  Differential Drive Kinematic Model1/1 -> x-y-yaw/1
  Differential Drive Kinematic Model1/2 -> dot/1

== system b6_formation/Subsystem1/car_model3 ==
  note: tr=0.6
      | 4T=0.6
      | 一阶系统的动态性能指标为：td=0.69T，tr=2.20T，ts=3T
  vw1 : Inport
  Demux : Demux  Outputs=2
  Differential Drive Kinematic Model1 : robotmobilelib/Differential Drive Kinematic Model  VehicleInputs=Vehicle Speed & Heading Angular Velocity  WheelRadius=wheelRadius  WheelSpeedRange=[-inf inf]  TrackWidth=robotRadius  InitialState=init_pose_3  SimulateUsing=Interpreted execution
      settings: SourceProductBaseCode=RO
  Simulink顺时针为正 小车逆时针为正 : Gain  Gain=ks
  Transfer Fcn : TransferFcn  Denominator=[0.15 1]
  Transfer Fcn1 : TransferFcn  Denominator=[0.16 1]
  x-y-yaw : Outport
  dot : Outport  Port=2
  wires:
  Simulink顺时针为正 小车逆时针为正/1 -> Transfer Fcn1/1
  Transfer Fcn/1 -> Differential Drive Kinematic Model1/1
  Demux/1 -> Transfer Fcn/1
  Transfer Fcn1/1 -> Differential Drive Kinematic Model1/2
  Demux/2 -> Simulink顺时针为正 小车逆时针为正/1
  vw1/1 -> Demux/1
  Differential Drive Kinematic Model1/1 -> x-y-yaw/1
  Differential Drive Kinematic Model1/2 -> dot/1

== system b6_formation/Subsystem1/car_model4 ==
  note: tr=0.6
      | 4T=0.6
      | 一阶系统的动态性能指标为：td=0.69T，tr=2.20T，ts=3T
  vw1 : Inport
  Demux : Demux  Outputs=2
  Differential Drive Kinematic Model1 : robotmobilelib/Differential Drive Kinematic Model  VehicleInputs=Vehicle Speed & Heading Angular Velocity  WheelRadius=wheelRadius  WheelSpeedRange=[-inf inf]  TrackWidth=robotRadius  InitialState=init_pose_4  SimulateUsing=Interpreted execution
      settings: SourceProductBaseCode=RO
  Simulink顺时针为正 小车逆时针为正 : Gain  Gain=ks
  Transfer Fcn : TransferFcn  Denominator=[0.15 1]
  Transfer Fcn1 : TransferFcn  Denominator=[0.16 1]
  x-y-yaw : Outport
  dot : Outport  Port=2
  wires:
  Simulink顺时针为正 小车逆时针为正/1 -> Transfer Fcn1/1
  Transfer Fcn/1 -> Differential Drive Kinematic Model1/1
  Demux/1 -> Transfer Fcn/1
  Transfer Fcn1/1 -> Differential Drive Kinematic Model1/2
  Demux/2 -> Simulink顺时针为正 小车逆时针为正/1
  vw1/1 -> Demux/1
  Differential Drive Kinematic Model1/1 -> x-y-yaw/1
  Differential Drive Kinematic Model1/2 -> dot/1

== system b6_formation/Subsystem1/car_model5 ==
  note: tr=0.6
      | 4T=0.6
      | 一阶系统的动态性能指标为：td=0.69T，tr=2.20T，ts=3T
  vw1 : Inport
  Demux : Demux  Outputs=2
  Differential Drive Kinematic Model1 : robotmobilelib/Differential Drive Kinematic Model  VehicleInputs=Vehicle Speed & Heading Angular Velocity  WheelRadius=wheelRadius  WheelSpeedRange=[-inf inf]  TrackWidth=robotRadius  InitialState=init_pose_5  SimulateUsing=Interpreted execution
      settings: SourceProductBaseCode=RO
  Simulink顺时针为正 小车逆时针为正 : Gain  Gain=ks
  Transfer Fcn : TransferFcn  Denominator=[0.15 1]
  Transfer Fcn1 : TransferFcn  Denominator=[0.16 1]
  x-y-yaw : Outport
  dot : Outport  Port=2
  wires:
  Simulink顺时针为正 小车逆时针为正/1 -> Transfer Fcn1/1
  Transfer Fcn/1 -> Differential Drive Kinematic Model1/1
  Demux/1 -> Transfer Fcn/1
  Transfer Fcn1/1 -> Differential Drive Kinematic Model1/2
  Demux/2 -> Simulink顺时针为正 小车逆时针为正/1
  vw1/1 -> Demux/1
  Differential Drive Kinematic Model1/1 -> x-y-yaw/1
  Differential Drive Kinematic Model1/2 -> dot/1

== system b6_formation/Subsystem1/car_model6 ==
  note: tr=0.6
      | 4T=0.6
      | 一阶系统的动态性能指标为：td=0.69T，tr=2.20T，ts=3T
  vw1 : Inport
  Demux : Demux  Outputs=2
  Differential Drive Kinematic Model1 : robotmobilelib/Differential Drive Kinematic Model  VehicleInputs=Vehicle Speed & Heading Angular Velocity  WheelRadius=wheelRadius  WheelSpeedRange=[-inf inf]  TrackWidth=robotRadius  InitialState=init_pose_6  SimulateUsing=Interpreted execution
      settings: SourceProductBaseCode=RO
  Simulink顺时针为正 小车逆时针为正 : Gain  Gain=ks
  Transfer Fcn : TransferFcn  Denominator=[0.15 1]
  Transfer Fcn1 : TransferFcn  Denominator=[0.16 1]
  x-y-yaw : Outport
  dot : Outport  Port=2
  wires:
  Simulink顺时针为正 小车逆时针为正/1 -> Transfer Fcn1/1
  Transfer Fcn/1 -> Differential Drive Kinematic Model1/1
  Demux/1 -> Transfer Fcn/1
  Transfer Fcn1/1 -> Differential Drive Kinematic Model1/2
  Demux/2 -> Simulink顺时针为正 小车逆时针为正/1
  vw1/1 -> Demux/1
  Differential Drive Kinematic Model1/1 -> x-y-yaw/1
  Differential Drive Kinematic Model1/2 -> dot/1

== system b6_formation/controller/Car1 ==
  Ranges : Inport
  Pose : Inport  Port=2
  WayPoints : Inport  Port=3
  Constant7 : Constant  Value=scanAngles
  Mux1 : Mux  Inputs=2
  ppCar : Subsystem
  Out1 : Outport
  wires:
  WayPoints/1 -> ppCar/4(WayPoints)
  Pose/1 -> ppCar/3(Pose)
  Ranges/1 -> ppCar/2(Ranges)
  ppCar/2(w) -> Mux1/2
  Mux1/1 -> Out1/1
  ppCar/1(v) -> Mux1/1
  Constant7/1 -> ppCar/1(Angels)

== system b6_formation/controller/Car2 ==
  Ranges : Inport
  Pose : Inport  Port=2
  WayPoints : Inport  Port=3
  Constant7 : Constant  Value=scanAngles
  Mux1 : Mux  Inputs=2
  ppCar : Subsystem
  Out1 : Outport
  wires:
  Constant7/1 -> ppCar/1(Angels)
  ppCar/1(v) -> Mux1/1
  Mux1/1 -> Out1/1
  ppCar/2(w) -> Mux1/2
  Ranges/1 -> ppCar/2(Ranges)
  Pose/1 -> ppCar/3(Pose)
  WayPoints/1 -> ppCar/4(WayPoints)

== system b6_formation/controller/Car3 ==
  Ranges : Inport
  Pose : Inport  Port=2
  WayPoints : Inport  Port=3
  Constant7 : Constant  Value=scanAngles
  Mux1 : Mux  Inputs=2
  ppCar : Subsystem
  Out1 : Outport
  wires:
  WayPoints/1 -> ppCar/4(WayPoints)
  Pose/1 -> ppCar/3(Pose)
  Ranges/1 -> ppCar/2(Ranges)
  ppCar/2(w) -> Mux1/2
  Mux1/1 -> Out1/1
  ppCar/1(v) -> Mux1/1
  Constant7/1 -> ppCar/1(Angels)

== system b6_formation/controller/Car4 ==
  Ranges : Inport
  Pose : Inport  Port=2
  WayPoints : Inport  Port=3
  Constant7 : Constant  Value=scanAngles
  Mux1 : Mux  Inputs=2
  ppCar : Subsystem
  Out1 : Outport
  wires:
  Constant7/1 -> ppCar/1(Angels)
  ppCar/1(v) -> Mux1/1
  Mux1/1 -> Out1/1
  ppCar/2(w) -> Mux1/2
  Ranges/1 -> ppCar/2(Ranges)
  Pose/1 -> ppCar/3(Pose)
  WayPoints/1 -> ppCar/4(WayPoints)

== system b6_formation/controller/Car5 ==
  Ranges : Inport
  Pose : Inport  Port=2
  WayPoints : Inport  Port=3
  Constant7 : Constant  Value=scanAngles
  Mux1 : Mux  Inputs=2
  ppCar : Subsystem
  Out1 : Outport
  wires:
  WayPoints/1 -> ppCar/4(WayPoints)
  Pose/1 -> ppCar/3(Pose)
  Ranges/1 -> ppCar/2(Ranges)
  ppCar/2(w) -> Mux1/2
  Mux1/1 -> Out1/1
  ppCar/1(v) -> Mux1/1
  Constant7/1 -> ppCar/1(Angels)

== system b6_formation/controller/Car6 ==
  Ranges : Inport
  Pose : Inport  Port=2
  WayPoints : Inport  Port=3
  Constant7 : Constant  Value=scanAngles
  Mux1 : Mux  Inputs=2
  ppCar : Subsystem
  Out1 : Outport
  wires:
  Constant7/1 -> ppCar/1(Angels)
  ppCar/1(v) -> Mux1/1
  Mux1/1 -> Out1/1
  ppCar/2(w) -> Mux1/2
  Ranges/1 -> ppCar/2(Ranges)
  Pose/1 -> ppCar/3(Pose)
  WayPoints/1 -> ppCar/4(WayPoints)

== system b6_formation/controller/controller1 ==
  poses : Inport
  Constant : Constant
  Constant1 : Constant  Value=2
  Constant2 : Constant  Value=3
  Constant3 : Constant  Value=4
  Constant4 : Constant  Value=5
  Constant5 : Constant  Value=6
  MATLAB Function1 : MATLAB Function  TreatAsAtomicUnit=on
  MATLAB Function10 : MATLAB Function  TreatAsAtomicUnit=on
  MATLAB Function2 : MATLAB Function  TreatAsAtomicUnit=on
  MATLAB Function3 : MATLAB Function  TreatAsAtomicUnit=on
  MATLAB Function4 : MATLAB Function  TreatAsAtomicUnit=on
  MATLAB Function5 : MATLAB Function  TreatAsAtomicUnit=on
  Reshape1 : Reshape  OutputDimensionality=Customize  OutputDimensions=[3,6]
  Lidar1 : Outport
  Lidar2 : Outport  Port=2
  Lidar3 : Outport  Port=3
  Lidar4 : Outport  Port=4
  Lidar5 : Outport  Port=5
  Lidar6 : Outport  Port=6
  wires:
  poses/1 -> Reshape1/1
  MATLAB Function10/1(ranges) -> Lidar1/1
  Constant/1 -> MATLAB Function10/2(idx)
  Constant1/1 -> MATLAB Function5/2(idx)
  Constant2/1 -> MATLAB Function1/2(idx)
  Reshape1/1 -> MATLAB Function5/1(poses), MATLAB Function1/1(poses), MATLAB Function2/1(poses), MATLAB Function3/1(poses), MATLAB Function4/1(poses), MATLAB Function10/1(poses)
  MATLAB Function5/1(ranges) -> Lidar2/1
  MATLAB Function1/1(ranges) -> Lidar3/1
  MATLAB Function2/1(ranges) -> Lidar4/1
  MATLAB Function3/1(ranges) -> Lidar5/1
  MATLAB Function4/1(ranges) -> Lidar6/1
  Constant3/1 -> MATLAB Function2/2(idx)
  Constant5/1 -> MATLAB Function4/2(idx)
  Constant4/1 -> MATLAB Function3/2(idx)
